simulink model "pfb_fir"  (Simulink 7.0)
settings: Solver=FixedStepDiscrete  SolverMode=SingleTasking  StartTime=0.0  StopTime=10.0  RelTol=1e-3
undefined symbols (not defined in the file): pfb_coefs
libraries: xbsIndex_r4 x385
(part 6 of 27)

== system pfb_fir/fir_1/fir_tap_4 ==
  data_in : Inport  OutDataType=sfix(16)  OutScaling=2^0
  sum_in : Inport  Port=2  OutDataType=sfix(16)  OutScaling=2^0
  sync_in : Inport  Port=3  OutDataType=sfix(16)  OutScaling=2^0
  fir_coef : Subsystem  mask(FIR Filter Coefficient Generator){coef=[0.000376226431598763;0.00113037704120664;0.00188679033646423;0.00264546512738635;0.00340640020282435;0.00416959433045314;0.00493504625675948;0.00570275470702945;0.00647271838533626;0.00724493597452914;0.00801940613622144;0.00879612751077952;0.00957509871731131;0.0103563183536561;0.0111397849963734;0.0119254972007329;0.0127134535007037;0.0135036524089452;0.0142960924167967;0.0150907719942678;0.0158876895900297;0.0166868436314057;0.0174882325243625;0.0182918546535009;0.0190977083820486;0.019905792051851;0.0207161039833637;0.0215286424756441;0.022343405806345;0.0231603922317064;0.0239795999865484;0.0248010272842649;0.0256246723168164;0.026450533254724;0.0272786082470629;0.0281088954214566;0.0289413928840709;0.0297760987196091;0.0306130109913055;0.0314521277409214;0.0322934469887399;0.0331369667335609;0.0339826849526973;0.0348305996019707;0.035680708615707;0.0365330099067331;0.0373875013663734;0.0382441808644464;0.0391030462492619;0.0399640953476175;0.0408273259647971;0.0416927358845677;0.0425603228691775;0.0434300846593541;0.0443020189743029;0.0451761235117054;0.0460523959477181;0.0469308339369715;0.0478114351125697;0.0486941970860893;0.0495791174475793;0.0504661937655611;0.0513554235870291;0.0522468044374499;0.0531403338207642;0.0540360092193872;0.0549338280942094;0.055833787884598;0.0567358860083988;0.0576401198619378;0.0585464868200229;0.0594549842359465;0.0603656094414881;0.0612783597469165;0.062193232440993;0.0631102247909746;0.0640293340426176;0.0649505574201807;0.0658738921264291;0.066799335342639;0.0677268842286013;0.0686565359226264;0.069588287541549;0.0705221361807334;0.0714580789140785;0.0723961127940227;0.0733362348515507;0.0742784420961991;0.0752227315160621;0.0761691000777984;0.0771175447266376;0.0780680623863875;0.0790206499594406;0.0799753043267821;0.0809320223479969;0.081890800861278;0.0828516366834338;0.0838145266098974;0.0847794674147343;0.0857464558506515;0.0867154886490061;0.0876865625198155;0.0886596741517658;0.0896348202122217;0.0906119973472373;0.091591202181565;0.0925724313186671;0.0935556813407251;0.094540948808652;0.0955282302621025;0.0965175222194845;0.0975088211779706;0.0985021236135104;0.0994974259808421;0.100494724713505;0.10149401622385;0.102495296903059;0.103498563121147;0.104503811226986;0.105511037548312;0.106520238391741;0.107531410042783;0.108544548765853;0.109559650804292;0.110576712380376;0.111595729695331;0.112616698929352;0.113639616241614;0.114664477770291;0.11569127963257;0.116720017924666;0.117750688721843;0.118783288078423;0.11981781202781;0.120854256582503;0.121892617734113;0.122932891453382;0.123975073690202;0.125019160373628;0.126065147411903;0.12711303069247;0.128162806081993;0.129214469426379;0.13026801655079;0.131323443259671;0.132380745336762;0.133439918545122;0.134500958627148;0.135563861304595;0.136628622278597;0.137695237229687;0.138763701817818;0.139834011682386;0.140906162442248;0.141980149695748;0.143055969020734;0.144133615974584;0.145213086094228;0.146294374896168;0.147377477876504;0.148462390510953;0.149549108254878;0.150637626543306;0.151727940790955;0.152820046392257;0.153913938721383;0.155009613132265;0.156107064958625;0.157206289513996;0.158307282091748;0.159410037965114;0.160514552387217;0.161620820591094;0.162728837789721;0.163838599176042;0.164950099922995;0.166063335183536;0.167178300090671;0.168294989757478;0.169413399277137;0.170533523722959;0.171655358148411;0.172778897587147;0.173904137053034;0.175031071540182;0.176159696022971;0.177290005456083;0.178421994774532;0.179555658893686;0.180690992709306;0.181827991097572;0.182966648915113;0.184106960999035;0.185248922166959;0.186392527217044;0.187537770928023;0.188684648059233;0.189833153350645;0.190983281522898;0.192135027277332;0.193288385296015;0.194443350241782;0.195599916758264;0.196758079469921;0.197917832982076;0.199079171880949;0.200242090733689;0.201406584088409;0.202572646474221;0.203740272401268;0.204909456360757;0.206080192825002;0.207252476247449;0.208426301062716;0.209601661686629 ...(+14467 chars)], n_bits_c=9, bin_pt_c=8, use_bram=on}
      mask prompts: coef "Tap Coefficient(s)"; n_bits_c "Number of Coefficient Bits"; bin_pt_c "Coefficient Binary Point"; use_bram "Use BRAM for Coefficients"
      mask help: A Finite Impluse Response filter coefficient generator. This FIR filter coefficient generator outputs real coefficients. It can output one coefficient or cycle through a vector of coefficients for WOLA (Weighted OverLap Add) FIR filters.
      settings: AttributesFormatString=1024 coefs in bram
      mask Help:
      | <pre>
      | Description::
      | 
      | A Finite Impluse Response filter coefficient generator.
      | This FIR filter coefficient generator outputs real coefficients.
      | It can output one coefficient or cycle through a vector of coefficients for WOLA
      | (Weighted OverLap Add) FIR filters.
      | 
      | Mask Parameters::
      | 
      | Tap Coefficiant(s) (coef): The coefficient(s) to output.  For a "regular" FIR filter, this will be a
      | single number.  For a WOLA (Weighted OverLap Add) filter, this will be a vector of numbers.
      | These should be specified as doubles.   They will be rounded and saturated according to the
      | specified number of bits (n_bits_c) and binary point (bin_pt_c).
      | 
      | Number of Coefficient Bits (n_bits_c): The number of bits used for the fixed point binary
      | representation of the coefficient(s).
      | 
      | Coefficient Binary Point (bin_pt_c): The binary point of the fixed point binary representation
      | of the coefficient(s).
      | 
      | Use BRAM for Coefficients (use_bram): Check this checkbox to store the coefficients in BRAM.
      | If unchecked, the coefficients will be stored in distributed memory (i.e. slices).
      | This is only relevant is length(coef) is greater than 1; otherwise, a constant block is used.
      | </pre>
  fir_core : Subsystem  mask(FIR Filter Core){delay=1024, n_bits_d=8, bin_pt_d=7, n_bits_s=17, bin_pt_s=15, use_bram=on, mult_latency=3, add_latency=1, add_bypass=off}
      mask prompts: delay "Tap Delay"; n_bits_d "Number of Data Bits"; bin_pt_d "Data Binary Point"; n_bits_s "Number of Sum Bits"; bin_pt_s "Sum Binary Point"; use_bram "Use BRAM for Delay"; mult_latency "Multiplier Latency"; add_latency "Adder Latency"; add_bypass "Bypass Adder"
      mask help: A Finite Impluse Response Filter core with complex inputs and real coefficients. This FIR filter core does not have provisions for folding the input sequence to improve multiplier efficiency, so it is suboptimal for "regular" (i.e. non-WOLA) FIR filters. It is intended primarily for WOLA (Weighted OverLap Add) FIR filters.
      settings: AttributesFormatString=delay 1024 in bram
      mask Help:
      | <pre>
      | Description::
      | 
      | A Finite Impluse Response Filter core with complex inputs and real coefficients.
      | 
      | This Finite Impluse Response Filter core is designed to be paired with a FIR Coefficient Generator
      | to form a FIR filter tap.  This FIR filter core does not have provisions for folding the input
      | sequence to improve multiplier efficiency, so it is suboptimal for "regular" (i.e. non-WOLA)
      | FIR filters.  It is intended primarily for WOLA (Weighted OverLap Add) FIR filters.
      | 
      | Mask Parameters::
      | 
      | Tap Delay (delay):  The inter-tap delay (the N in "z^-N").  For a regular FIR filter, this will be 1.
      | 
      | Number of Data Bits (n_bits_d): The number of bits for real/imaginary components of the data.
      | 
      | Data Binary Point (bin_pt_d): The binary point for real/imaginary components of the data.
      | 
      | Number of Sum Bits (n_bits_s): Specifies the width of the sum (overflow wraps).
      | 
      | Sum Binary Point (bin_pt_s): Specifies the binary point of the sum (quantization truncates).
      | 
      | Use BRAM for Delay (use_bram): Check this checkbox to implement the delay using BRAM.
      | If unchecked, the delay will be implemented using SLR16 elements (i.e. slices).
      | 
      | Multiplier Latency (mult_latency): Latency to use for the underlying multiplier.
      | 
      | Adder Latency (add_latency): Latency to use for the underlying adder.
      | 
      | Adder Bypass (add_bypass): Check this checkbox to bypass the adder.
      | Typically used for the first tap of a multi-tap FIR filter.
      | </pre>
  data_out : Outport  OutDataType=sfix(16)  OutScaling=2^0
  sum_out : Outport  Port=2  OutDataType=sfix(16)  OutScaling=2^0
  sync_out : Outport  Port=3  OutDataType=sfix(16)  OutScaling=2^0
  wires:
  fir_core/3(sync_out) -> sync_out/1
  fir_core/2(sum_out) -> sum_out/1
  fir_core/1(data_out) -> data_out/1
  sync_in/1 -> fir_coef/3(sync_in)
  sum_in/1 -> fir_coef/2(sum_in)
  data_in/1 -> fir_coef/1(data_in)
  fir_coef/4(sync_out) -> fir_core/4(sync_in)
  fir_coef/3(coef) -> fir_core/3(coef)
  fir_coef/2(sum_out) -> fir_core/2(sum_in)
  fir_coef/1(data_out) -> fir_core/1(data_in)

== system pfb_fir/fir_1/fir_tap_5 ==
  data_in : Inport  OutDataType=sfix(16)  OutScaling=2^0
  sum_in : Inport  Port=2  OutDataType=sfix(16)  OutScaling=2^0
  sync_in : Inport  Port=3  OutDataType=sfix(16)  OutScaling=2^0
  fir_coef : Subsystem  mask(FIR Filter Coefficient Generator){coef=[-7.57186305694141e-005;-0.000227564945670749;-0.000379956430889435;-0.000532892796251757;-0.000686373742881339;-0.000840398962979647;-0.000994968139806186;-0.00115008094765919;-0.00130573705185642;-0.00146193610871559;-0.00161867776553536;-0.00177596166057639;-0.00193378742304204;-0.0020921546730598;-0.0022510630216622;-0.00241051207076825;-0.00257050141316491;-0.00273103063248833;-0.00289209930320557;-0.00305370699059638;-0.00321585325073467;-0.00337853763047057;-0.00354175966741245;-0.00370551888990871;-0.00386981481703025;-0.00403464695855241;-0.00420001481493748;-0.00436591787731722;-0.0045323556274752;-0.00469932753782952;-0.00486683307141569;-0.00503487168186923;-0.00520344281340873;-0.00537254590081901;-0.00554218036943399;-0.00571234563512023;-0.00588304110426002;-0.00605426617373492;-0.00622602023090949;-0.00639830265361464;-0.00657111281013151;-0.00674445005917552;-0.00691831374988003;-0.00709270322178053;-0.00726761780479901;-0.00744305681922785;-0.00761901957571464;-0.00779550537524631;-0.0079725135091339;-0.00815004325899737;-0.00832809389675017;-0.0085066646845843;-0.00868575487495546;-0.00886536371056795;-0.00904549042435999;-0.00922613423948933;-0.00940729436931827;-0.0095889700173997;-0.00977116037746245;-0.00995386463339719;-0.0101370819592425;-0.0103208115191707;-0.010505052467474;-0.0106898039485508;-0.0108750650968923;-0.0110608350370682;-0.0112471128837145;-0.011433897741519;-0.0116211887052088;-0.0118089848595372;-0.0119972852792704;-0.0121860890291751;-0.0123753951640054;-0.0125652027284904;-0.0127555107573218;-0.0129463182751411;-0.013137624296528;-0.0133294278259877;-0.0135217278579391;-0.013714523376703;-0.0139078133564902;-0.0141015967613896;-0.0142958725453573;-0.0144906396522044;-0.0146858970155864;-0.0148816435589916;-0.01507787819573;-0.0152745998289226;-0.0154718073514906;-0.0156694996461444;-0.0158676755853733;-0.016066334031435;-0.016265473836345;-0.0164650938418669;-0.016665192879502;-0.0168657697704791;-0.0170668233257453;-0.0172683523459559;-0.0174703556214645;-0.0176728319323143;-0.0178757800482282;-0.0180791987285998;-0.0182830867224842;-0.018487442768589;-0.0186922655952659;-0.0188975539205014;-0.0191033064519087;-0.019309521886719;-0.0195161989117731;-0.0197233362035136;-0.0199309324279764;-0.0201389862407831;-0.020347496287133;-0.0205564612017955;-0.0207658796091025;-0.0209757501229411;-0.0211860713467461;-0.0213968418734932;-0.0216080602856917;-0.0218197251553776;-0.022031835044107;-0.0222443885029495;-0.0224573840724814;-0.0226708202827797;-0.0228846956534157;-0.0230990086934489;-0.0233137579014212;-0.0235289417653507;-0.0237445587627263;-0.0239606073605024;-0.0241770860150929;-0.024393993172366;-0.0246113272676396;-0.0248290867256759;-0.025047269960676;-0.0252658753762764;-0.0254849013655432;-0.0257043463109681;-0.0259242085844644;-0.026144486547362;-0.0263651785504042;-0.026586282933743;-0.026807798026936;-0.0270297221489423;-0.0272520536081191;-0.0274747907022183;-0.0276979317183836;-0.0279214749331467;-0.0281454186124251;-0.0283697610115189;-0.0285945003751079;-0.0288196349372498;-0.029045162921377;-0.0292710825402948;-0.0294973919961793;-0.0297240894805752;-0.0299511731743939;-0.0301786412479123;-0.0304064918607708;-0.0306347231619722;-0.03086333328988;-0.0310923203722177;-0.0313216825260677;-0.0315514178578704;-0.0317815244634236;-0.0320120004278819;-0.0322428438257562;-0.0324740527209136;-0.0327056251665774;-0.0329375592053265;-0.0331698528690966;-0.0334025041791795;-0.0336355111462241;-0.0338688717702371;-0.0341025840405833;-0.0343366459359869;-0.0345710554245323;-0.0348058104636656;-0.0350409090001953;-0.0352763489702948;-0.035512128299503;-0.0357482449027266;-0.0359846966842419;-0.036221481537697;-0.036458597346114;-0.0366960419818909;-0.0369338133068049;-0.0371719091720144;-0.0374103274180622;-0.037649065874878;-0.0378881223617824;-0.038127494687489;-0.0383671806501086;-0.0386071780371525;-0.0388474846255361;-0.0390880981815831;-0.039329016461029;-0.0395702372090256 ...(+16053 chars)], n_bits_c=9, bin_pt_c=8, use_bram=on}
      mask prompts: coef "Tap Coefficient(s)"; n_bits_c "Number of Coefficient Bits"; bin_pt_c "Coefficient Binary Point"; use_bram "Use BRAM for Coefficients"
      mask help: A Finite Impluse Response filter coefficient generator. This FIR filter coefficient generator outputs real coefficients. It can output one coefficient or cycle through a vector of coefficients for WOLA (Weighted OverLap Add) FIR filters.
      settings: AttributesFormatString=1024 coefs in bram
      mask Help:
      | <pre>
      | Description::
      | 
      | A Finite Impluse Response filter coefficient generator.
      | This FIR filter coefficient generator outputs real coefficients.
      | It can output one coefficient or cycle through a vector of coefficients for WOLA
      | (Weighted OverLap Add) FIR filters.
      | 
      | Mask Parameters::
      | 
      | Tap Coefficiant(s) (coef): The coefficient(s) to output.  For a "regular" FIR filter, this will be a
      | single number.  For a WOLA (Weighted OverLap Add) filter, this will be a vector of numbers.
      | These should be specified as doubles.   They will be rounded and saturated according to the
      | specified number of bits (n_bits_c) and binary point (bin_pt_c).
      | 
      | Number of Coefficient Bits (n_bits_c): The number of bits used for the fixed point binary
      | representation of the coefficient(s).
      | 
      | Coefficient Binary Point (bin_pt_c): The binary point of the fixed point binary representation
      | of the coefficient(s).
      | 
      | Use BRAM for Coefficients (use_bram): Check this checkbox to store the coefficients in BRAM.
      | If unchecked, the coefficients will be stored in distributed memory (i.e. slices).
      | This is only relevant is length(coef) is greater than 1; otherwise, a constant block is used.
      | </pre>
  fir_core : Subsystem  mask(FIR Filter Core){delay=1024, n_bits_d=8, bin_pt_d=7, n_bits_s=17, bin_pt_s=15, use_bram=on, mult_latency=3, add_latency=1, add_bypass=off}
      mask prompts: delay "Tap Delay"; n_bits_d "Number of Data Bits"; bin_pt_d "Data Binary Point"; n_bits_s "Number of Sum Bits"; bin_pt_s "Sum Binary Point"; use_bram "Use BRAM for Delay"; mult_latency "Multiplier Latency"; add_latency "Adder Latency"; add_bypass "Bypass Adder"
      mask help: A Finite Impluse Response Filter core with complex inputs and real coefficients. This FIR filter core does not have provisions for folding the input sequence to improve multiplier efficiency, so it is suboptimal for "regular" (i.e. non-WOLA) FIR filters. It is intended primarily for WOLA (Weighted OverLap Add) FIR filters.
      settings: AttributesFormatString=delay 1024 in bram
      mask Help:
      | <pre>
      | Description::
      | 
      | A Finite Impluse Response Filter core with complex inputs and real coefficients.
      | 
      | This Finite Impluse Response Filter core is designed to be paired with a FIR Coefficient Generator
      | to form a FIR filter tap.  This FIR filter core does not have provisions for folding the input
      | sequence to improve multiplier efficiency, so it is suboptimal for "regular" (i.e. non-WOLA)
      | FIR filters.  It is intended primarily for WOLA (Weighted OverLap Add) FIR filters.
      | 
      | Mask Parameters::
      | 
      | Tap Delay (delay):  The inter-tap delay (the N in "z^-N").  For a regular FIR filter, this will be 1.
      | 
      | Number of Data Bits (n_bits_d): The number of bits for real/imaginary components of the data.
      | 
      | Data Binary Point (bin_pt_d): The binary point for real/imaginary components of the data.
      | 
      | Number of Sum Bits (n_bits_s): Specifies the width of the sum (overflow wraps).
      | 
      | Sum Binary Point (bin_pt_s): Specifies the binary point of the sum (quantization truncates).
      | 
      | Use BRAM for Delay (use_bram): Check this checkbox to implement the delay using BRAM.
      | If unchecked, the delay will be implemented using SLR16 elements (i.e. slices).
      | 
      | Multiplier Latency (mult_latency): Latency to use for the underlying multiplier.
      | 
      | Adder Latency (add_latency): Latency to use for the underlying adder.
      | 
      | Adder Bypass (add_bypass): Check this checkbox to bypass the adder.
      | Typically used for the first tap of a multi-tap FIR filter.
      | </pre>
  data_out : Outport  OutDataType=sfix(16)  OutScaling=2^0
  sum_out : Outport  Port=2  OutDataType=sfix(16)  OutScaling=2^0
  sync_out : Outport  Port=3  OutDataType=sfix(16)  OutScaling=2^0
  wires:
  fir_core/3(sync_out) -> sync_out/1
  fir_core/2(sum_out) -> sum_out/1
  fir_core/1(data_out) -> data_out/1
  sync_in/1 -> fir_coef/3(sync_in)
  sum_in/1 -> fir_coef/2(sum_in)
  data_in/1 -> fir_coef/1(data_in)
  fir_coef/4(sync_out) -> fir_core/4(sync_in)
  fir_coef/3(coef) -> fir_core/3(coef)
  fir_coef/2(sum_out) -> fir_core/2(sum_in)
  fir_coef/1(data_out) -> fir_core/1(data_in)
